simulink model "Main"  (R2024a)
settings: Solver=VariableStepAuto  StartTime=0.0  StopTime=150  RelTol=1e-3
values from neighbouring files (symbols this model uses):
  controller = optimizer(constraints, objective,[],{x{1},r,Ad_,Bd_},[u{:}])    [MPC_Script.m]
  Ka = 1/(Ki*ts/3)    (= 0.15)    [Main_Script.m]
  Ki = 200    [Main_Script.m]
  Kp = 1500    [Main_Script.m]
  Psi0 = 245*pi/180    (= 4.27605666739)    [Main_Script.m]
  Ts = 0.01    [MPC_Script.m]    (also in MPC_Sim.m)
  X0 = 0    [Main_Script.m]
  Y0 = 0    [Main_Script.m]
undefined symbols (not defined in the file or in its folder): AdaptivepurePursuitRefGen, Kinematic_Model, LongDyn, Mapping_Fx_to_w, MPC_Sim, purePursuitRefGen, Track
settings Model: Creator=bensalso  LastModifiedBy=etudiant
settings SolverCC: AlgebraicLoopSolver=TrustRegion
settings DebuggingCC: UnconnectedInputMsg=warning  UnconnectedOutputMsg=warning  UnconnectedLineMsg=warning  ArithmeticOperatorsInVariantConditions=warning
settings ModelReferenceCC: EnableRefExpFcnMdlSchedulingChecks=on
settings SFSimCC: CustomCodeUndefinedFunction=UseInterfaceOnly
settings RTWCC: GPUComputeCapability=3.5  DLArmComputeVersion=19.05

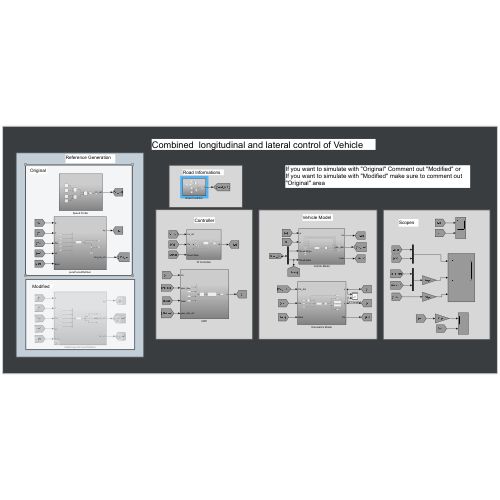
[thumbnail: Simulink's stored preview of the top-level diagram]
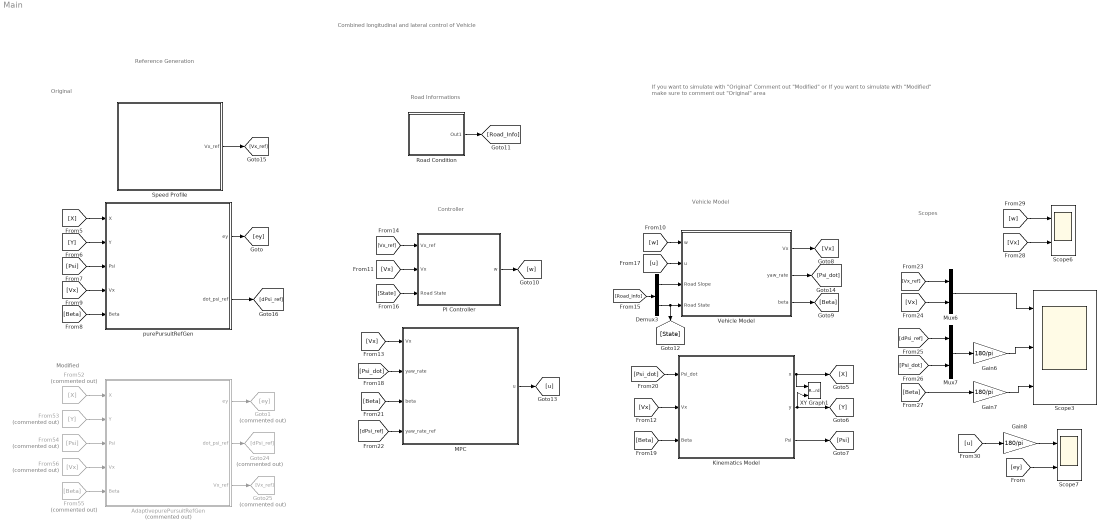
== system Main ==
  note: Combined longitudinal and lateral control of Vehicle
  note: If you want to simulate with "Original" Comment out "Modified" or
      | If you want to simulate with "Modified" make sure to comment out
      | "Original" area
  note: Modified
  note: Original
  note: Reference Generation
  note: Scopes
  note: Controller
  note: Vehicle Model
  note: Road Informations
  AdaptivepurePursuitRefGen : Subsystem  Commented=on
  Demux3 : Demux  Outputs=2
  From52 : From  Commented=on  GotoTag=X
  From53 : From  Commented=on  GotoTag=Y
  From54 : From  Commented=on  GotoTag=Psi
  From55 : From  Commented=on  GotoTag=Beta
  From56 : From  Commented=on  GotoTag=Vx
  Gain6 : Gain  Gain=180/pi
  Gain7 : Gain  Gain=180/pi
  Gain8 : Gain  Gain=180/pi
  Goto1 : Goto  Commented=on  GotoTag=ey
  Goto24 : Goto  Commented=on  GotoTag=dPsi_ref
  Goto25 : Goto  Commented=on  GotoTag=Vx_ref
  Kinematics Model : Subsystem
  MPC : Subsystem
  Mux6 : Mux  Inputs=2
  Mux7 : Mux  Inputs=2
  PI Controller : Subsystem
  Road Condition : Subsystem
  Scope3 : Scope  NumInputPorts=3
  Scope6 : Scope  NumInputPorts=2
  Scope7 : Scope  NumInputPorts=2
  "Speed Profile " : Subsystem
  Vehicle Model : Subsystem
  XY Graph1 : Record  FileSettingsInternal="{\"entries\":[{\"content\":{\"excelSettings\":{\"content\":{},\"type\":\"Streamout.ExcelSettings\"}},\"type\":\"Streamout.FileSettingStorage\",\"uuid\":\"\"}],\"packageUris\":[\"http:\\/\\/schema.mathworks.com\\/mf0\\/streamout_blocks\\/R2020a\"],\"version\":\"1.0\"}"  Layout=[1 1]  SignalsInternal="{\"entries\":[{\"content\":{\"signals\":[{\"content\":{\"blockPath\":[],\"dimensions\":[1],\"domain\":\"\",\"lineColor\":\"#a2142f\",\"plots\":[ 1 ],\"port\":1,\"sid\":[\"\"],\"signalID\":1,\"signalName\":\"Kinematics Model:1\"},\"type\":\"RecordBlkView.Signal\",\"uuid\":\"\"},{\"content\":{\"blockPath\":[],\"dimensions\":[1],\"domain\":\"\",\"lineColor\":\"#139fff\",\"plots\":[ 1 ],\"port\":2,\"sid\":[\"\"],\"signalID\":2,\"signalName\":\"Kinematics Model:2\"},\"type\":\"RecordBlkView.Signal\",\"uuid\":\"\"}]},\"type\":\"RecordBlkView.InputSignals\",\"uuid\":\"\"}],\"packageUris\":[\"http:\\/\\/schema.mathworks.com\\/mf0\\/streamout_blocks\\/R2020a\"],\"version\":\"1.0\"}"  VisualizationBindings="{\"xyplotplugin\":{\"info\":[{\"series\":[{\"bindingParametersList\":[{\"parameter\":\"X-Axis\",\"signalID\":1,\"signalName\":\"Kinematics Model:1\"},{\"parameter\":\"Y-Axis\",\"signalID\":2,\"signalName\":\"Kinematics Model:2\"}],\"seriesID\":0}],\"subplotID\":1}]}}"  CompatibilityTag=XY  st=-1
  purePursuitRefGen : Subsystem
  wires:
  [X] -> purePursuitRefGen/1(X)
  [Y] -> purePursuitRefGen/2(Y)
  [Psi] -> purePursuitRefGen/3(Psi)
  [Vx] -> purePursuitRefGen/4(Vx)
  [Beta] -> purePursuitRefGen/5(Beta)
  purePursuitRefGen/1(ey) -> [ey]
  MPC/1(u) -> [u]
  Vehicle Model/1(Vx) -> [Vx]
  Vehicle Model/2(yaw_rate) -> [Psi_dot]
  Vehicle Model/3(beta) -> [Beta]
  [w] -> Vehicle Model/1(w)
  PI Controller/1(w) -> [w]
  [Vx] -> PI Controller/2(Vx)
  [Vx] -> MPC/1(Vx)
  Road Condition/1(Out1) -> [Road_Info]
  [Road_Info] -> Demux3/1
  Demux3/1 -> Vehicle Model/3(Road Slope)
  Demux3/2 -> [State], Vehicle Model/4(Road State)
  [State] -> PI Controller/3(Road State)
  [u] -> Vehicle Model/2(u)
  [Psi_dot] -> MPC/2(yaw_rate)
  [Beta] -> MPC/3(beta)
  Kinematics Model/1(x) -> [X], XY Graph1/1
  Kinematics Model/2(y) -> [Y], XY Graph1/2
  [Psi_dot] -> Kinematics Model/1(Psi_dot)
  [Vx] -> Kinematics Model/2(Vx)
  [Beta] -> Kinematics Model/3(Beta)
  Kinematics Model/3(Psi) -> [Psi]
  "Speed Profile "/1(Vx_ref) -> [Vx_ref]
  [Vx_ref] -> PI Controller/1(Vx_ref)
  [dPsi_ref] -> MPC/4(yaw_rate_ref)
  purePursuitRefGen/2(dot_psi_ref) -> [dPsi_ref]
  Mux7/1 -> Gain6/1
  [Vx_ref] -> Mux6/1
  [Vx] -> Mux6/2
  [dPsi_ref] -> Mux7/1
  [Psi_dot] -> Mux7/2
  Mux6/1 -> Scope3/1
  Gain6/1 -> Scope3/2
  Gain7/1 -> Scope3/3
  [Beta] -> Gain7/1
  [w] -> Scope6/1
  [Vx] -> Scope6/2
  [u] -> Gain8/1
  Gain8/1 -> Scope7/1
  AdaptivepurePursuitRefGen/2(dot_psi_ref) -> Goto24/1
  AdaptivepurePursuitRefGen/3(Vx_ref) -> Goto25/1
  From52/1 -> AdaptivepurePursuitRefGen/1(X)
  AdaptivepurePursuitRefGen/1(ey) -> Goto1/1
  From55/1 -> AdaptivepurePursuitRefGen/5(Beta)
  From53/1 -> AdaptivepurePursuitRefGen/2(Y)
  From56/1 -> AdaptivepurePursuitRefGen/4(Vx)
  From54/1 -> AdaptivepurePursuitRefGen/3(Psi)
  [ey] -> Scope7/2

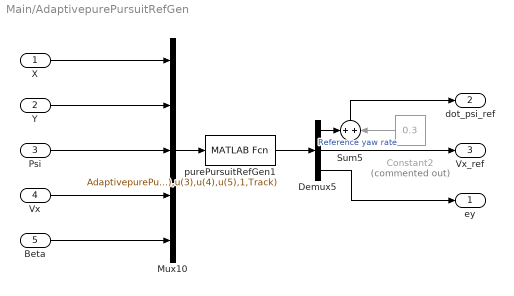
== system Main/AdaptivepurePursuitRefGen ==
  X : Inport
  Y : Inport  Port=2
  Psi : Inport  Port=3
  Vx : Inport  Port=4
  Beta : Inport  Port=5
  Constant2 : Constant  Commented=on  Value=0.3
  Demux5 : Demux  Outputs=3
  Mux10 : Mux  Inputs=5
  Sum5 : Sum
  purePursuitRefGen1 : MATLABFcn  MATLABFcn=AdaptivepurePursuitRefGen(u(1),u(2),u(3),u(4),u(5),1,Track)  OutputDimensions=3
  ey : Outport
  dot_psi_ref : Outport  Port=2
  Vx_ref : Outport  Port=3
  wires:
  Constant2/1 -> Sum5/2
  Mux10/1 -> purePursuitRefGen1/1
  purePursuitRefGen1/1 -> Demux5/1
  Sum5/1 -> dot_psi_ref/1
  X/1 -> Mux10/1
  Y/1 -> Mux10/2
  Psi/1 -> Mux10/3
  Vx/1 -> Mux10/4
  Beta/1 -> Mux10/5
  Demux5/3 -> ey/1
  Demux5/1 -> Sum5/1
  Demux5/2 -> Vx_ref/1  "Reference yaw rate"

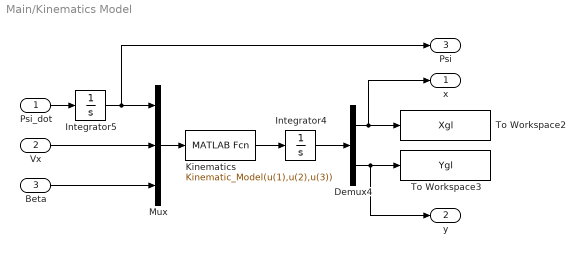
== system Main/Kinematics Model ==
  Psi_dot : Inport
  Vx : Inport  Port=2
  Beta : Inport  Port=3
  Demux4 : Demux  Outputs=2
  Integrator4 : Integrator  InitialCondition=[X0, Y0]
  Integrator5 : Integrator  InitialCondition=Psi0
  "Kinematics " : MATLABFcn  MATLABFcn=Kinematic_Model(u(1),u(2),u(3))  OutputDimensions=2
  Mux : Mux  Inputs=3
  To Workspace2 : ToWorkspace  VariableName=Xgl  SampleTime=-1
      settings: Save2DSignal=2-D array (concatenate along first dimension)
  To Workspace3 : ToWorkspace  VariableName=Ygl  SampleTime=-1
      settings: Save2DSignal=2-D array (concatenate along first dimension)
  x : Outport
  y : Outport  Port=2
  Psi : Outport  Port=3
  wires:
  Beta/1 -> Mux/3
  Demux4/2 -> y/1, To Workspace3/1
  Demux4/1 -> x/1, To Workspace2/1
  Integrator4/1 -> Demux4/1
  Vx/1 -> Mux/2
  "Kinematics "/1 -> Integrator4/1
  Integrator5/1 -> Mux/1, Psi/1
  Psi_dot/1 -> Integrator5/1
  Mux/1 -> "Kinematics "/1

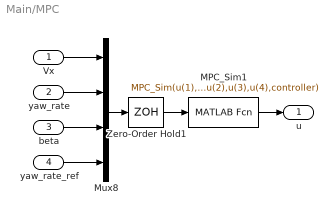
== system Main/MPC ==
  Vx : Inport
  yaw_rate : Inport  Port=2
  beta : Inport  Port=3
  yaw_rate_ref : Inport  Port=4
  MPC_Sim1 : MATLABFcn  MATLABFcn=MPC_Sim(u(1),u(2),u(3),u(4),controller)  OutputDimensions=1
  Mux8 : Mux
  Zero-Order Hold1 : ZeroOrderHold  SampleTime=Ts
  u : Outport
  wires:
  Mux8/1 -> Zero-Order Hold1/1
  MPC_Sim1/1 -> u/1
  Zero-Order Hold1/1 -> MPC_Sim1/1
  Vx/1 -> Mux8/1
  yaw_rate/1 -> Mux8/2
  beta/1 -> Mux8/3
  yaw_rate_ref/1 -> Mux8/4

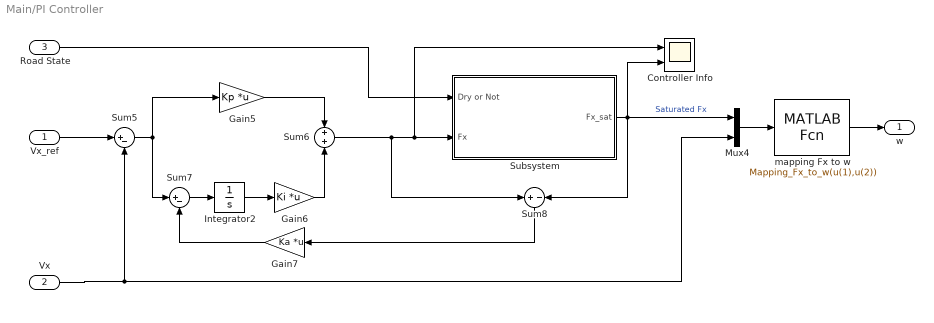
== system Main/PI Controller ==
  Vx_ref : Inport
  Vx : Inport  Port=2
  Road State : Inport  Port=3
  Controller Info : Scope  NumInputPorts=2
  Gain5 : Gain  Gain=Kp  Multiplication=Matrix(K*u)
  Gain6 : Gain  Gain=Ki  Multiplication=Matrix(K*u)
  Gain7 : Gain  Gain=Ka  Multiplication=Matrix(K*u)
  Integrator2 : Integrator  InitialCondition=0.1
  Mux4 : Mux  Inputs=2
  Subsystem : Subsystem
  Sum5 : Sum  Inputs=|+-
  Sum6 : Sum
  Sum7 : Sum  Inputs=|+-
  Sum8 : Sum  Inputs=+-
  mapping Fx to w : MATLABFcn  MATLABFcn=Mapping_Fx_to_w(u(1),u(2))  OutputDimensions=1
  w : Outport  VectorParamsAs1DForOutWhenUnconnected=off
  wires:
  Mux4/1 -> mapping Fx to w/1
  Subsystem/1(Fx_sat) -> Sum8/2, Mux4/1, Controller Info/2  "Saturated Fx"
  Sum6/1 -> Subsystem/2(Fx), Controller Info/1, Sum8/1
  Integrator2/1 -> Gain6/1
  Gain7/1 -> Sum7/2
  Road State/1 -> Subsystem/1(Dry or Not)
  Sum8/1 -> Gain7/1
  Vx/1 -> Mux4/2, Sum5/2
  Sum5/1 -> Gain5/1, Sum7/1
  Sum7/1 -> Integrator2/1
  mapping Fx to w/1 -> w/1
  Vx_ref/1 -> Sum5/1
  Gain5/1 -> Sum6/1
  Gain6/1 -> Sum6/2

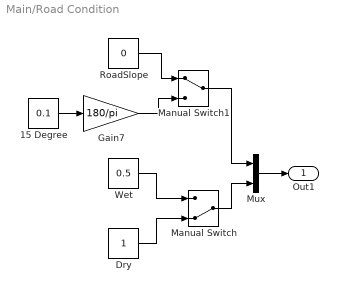
== system Main/Road Condition ==
  15 Degree : Constant  Value=0.1
  Dry : Constant
  Gain7 : Gain  Gain=180/pi
  Manual Switch : ManualSwitch  CurrentSetting=0
  Manual Switch1 : ManualSwitch
  Mux : Mux  Inputs=2
  RoadSlope : Constant  Value=0
  Wet : Constant  Value=0.5
  Out1 : Outport
  wires:
  Dry/1 -> Manual Switch/2
  Wet/1 -> Manual Switch/1
  Manual Switch/1 -> Mux/2
  Mux/1 -> Out1/1
  15 Degree/1 -> Gain7/1
  Manual Switch1/1 -> Mux/1
  RoadSlope/1 -> Manual Switch1/1
  Gain7/1 -> Manual Switch1/2

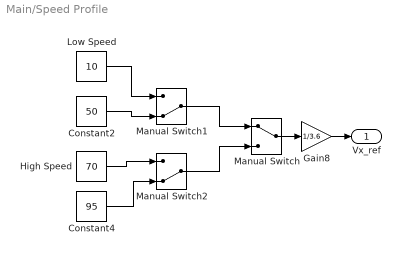
== system Main/Speed Profile  ==
  Constant2 : Constant  Value=50
  Constant4 : Constant  Value=95
  Gain8 : Gain  Gain=1/3.6
  High Speed : Constant  Value=70
  Low Speed : Constant  Value=10
  Manual Switch : ManualSwitch
  Manual Switch1 : ManualSwitch  CurrentSetting=0
  Manual Switch2 : ManualSwitch  CurrentSetting=0
  Vx_ref : Outport
  wires:
  Manual Switch2/1 -> Manual Switch/2
  Manual Switch/1 -> Gain8/1
  Manual Switch1/1 -> Manual Switch/1
  Constant4/1 -> Manual Switch2/2
  Low Speed/1 -> Manual Switch1/1
  High Speed/1 -> Manual Switch2/1
  Constant2/1 -> Manual Switch1/2
  Gain8/1 -> Vx_ref/1

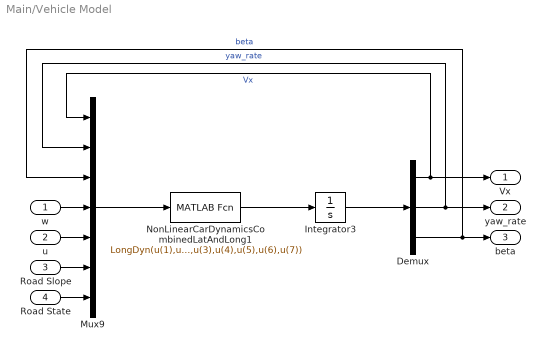
== system Main/Vehicle Model ==
  w : Inport
  u : Inport  Port=2
  Road Slope : Inport  Port=3
  Road State : Inport  Port=4
  Demux : Demux  Outputs=3
  Integrator3 : Integrator  InitialCondition=[20 ; 0; 0]
  Mux9 : Mux  Inputs=7
  NonLinearCarDynamicsCombinedLatAndLong1 : MATLABFcn  MATLABFcn=LongDyn(u(1),u(2),u(3),u(4),u(5),u(6),u(7))  OutputDimensions=3
  Vx : Outport
  yaw_rate : Outport  Port=2
  beta : Outport  Port=3
  wires:
  NonLinearCarDynamicsCombinedLatAndLong1/1 -> Integrator3/1
  Mux9/1 -> NonLinearCarDynamicsCombinedLatAndLong1/1
  u/1 -> Mux9/5
  w/1 -> Mux9/4
  Integrator3/1 -> Demux/1
  Demux/1 -> Mux9/1, Vx/1  "Vx"
  Demux/2 -> yaw_rate/1, Mux9/2  "yaw_rate"
  Demux/3 -> Mux9/3, beta/1  "beta"
  Road Slope/1 -> Mux9/6
  Road State/1 -> Mux9/7

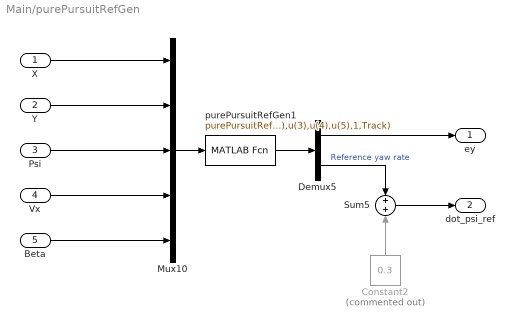
== system Main/purePursuitRefGen ==
  X : Inport
  Y : Inport  Port=2
  Psi : Inport  Port=3
  Vx : Inport  Port=4
  Beta : Inport  Port=5
  Constant2 : Constant  Commented=on  Value=0.3
  Demux5 : Demux  Outputs=2
  Mux10 : Mux  Inputs=5
  Sum5 : Sum
  purePursuitRefGen1 : MATLABFcn  MATLABFcn=purePursuitRefGen(u(1),u(2),u(3),u(4),u(5),1,Track)  OutputDimensions=2
  ey : Outport
  dot_psi_ref : Outport  Port=2
  wires:
  Constant2/1 -> Sum5/2
  Mux10/1 -> purePursuitRefGen1/1
  purePursuitRefGen1/1 -> Demux5/1
  Sum5/1 -> dot_psi_ref/1
  X/1 -> Mux10/1
  Y/1 -> Mux10/2
  Psi/1 -> Mux10/3
  Vx/1 -> Mux10/4
  Beta/1 -> Mux10/5
  Demux5/1 -> ey/1
  Demux5/2 -> Sum5/1  "Reference yaw rate"

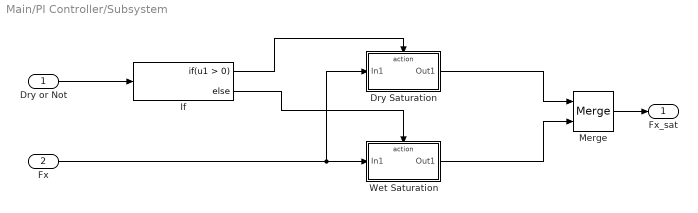
== system Main/PI Controller/Subsystem ==
  Dry or Not : Inport
  Fx : Inport  Port=2
  Dry Saturation : Subsystem  TreatAsAtomicUnit=on
  If : If
  Merge : Merge  InitialOutput=[0]
  Wet Saturation : Subsystem  TreatAsAtomicUnit=on
  Fx_sat : Outport  VectorParamsAs1DForOutWhenUnconnected=off
  wires:
  Wet Saturation/1(Out1) -> Merge/2
  Merge/1 -> Fx_sat/1
  Fx/1 -> Dry Saturation/1(In1), Wet Saturation/1(In1)
  Dry Saturation/1(Out1) -> Merge/1
  If/1 -> Dry Saturation/Action
  Dry or Not/1 -> If/1
  If/2 -> Wet Saturation/Action

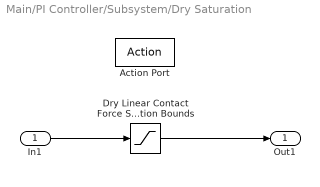
== system Main/PI Controller/Subsystem/Dry Saturation ==
  In1 : Inport
  Action Port : ActionPort  ActionPortLabel=if(u1 > 0)
  Dry Linear Contact Force Saturation Bounds : Saturate  UpperLimit=9000  LowerLimit=-9000
  Out1 : Outport  VectorParamsAs1DForOutWhenUnconnected=off
  wires:
  In1/1 -> Dry Linear Contact Force Saturation Bounds/1
  Dry Linear Contact Force Saturation Bounds/1 -> Out1/1

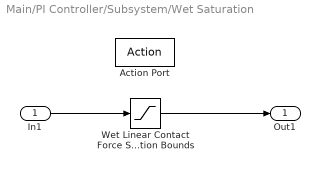
== system Main/PI Controller/Subsystem/Wet Saturation ==
  In1 : Inport
  Action Port : ActionPort  ActionPortLabel=else
  Wet Linear Contact Force Saturation Bounds : Saturate  UpperLimit=5000  LowerLimit=-5000
  Out1 : Outport  VectorParamsAs1DForOutWhenUnconnected=off
  wires:
  In1/1 -> Wet Linear Contact Force Saturation Bounds/1
  Wet Linear Contact Force Saturation Bounds/1 -> Out1/1
